simulink model "pixhawk_controller_position__ptCloud4_1"  (R2020a)
settings: Solver=ode4  StartTime=0.0  StopTime=30  FixedStep=0.01  RelTol=1e-3  EnableMultiTasking=on
InitFcn:
  | detector = load('ptOPDetector.mat');
  | OPdetector = detector.OPdetector;
undefined symbols (not defined in the file): g, Kd_p, Kd_q, Kd_r, Kd_vx, Kd_vy, Kd_vz, Kff_r, Kff_vx, Kff_vy, Kff_vz, Ki_p, Ki_q, Ki_r, Ki_vx, Ki_vy, Ki_vz, Kp_p, Kp_phi, Kp_psi, Kp_q, Kp_r, Kp_theta, Kp_vx, Kp_vy, Kp_vz, M, pointCloud_center, sigma_motor, w_h
libraries: visiontextngfix x1, sharedtransform x1, shared6dof x1, simulink_extras x1
(part 2 of 2)

== matlab function pixhawk_controller_position__ptCloud4_1/3D A* Algorithm/MATLAB Function8 ==
  data: octomap_center input; Obstacle output; pos_init input
function Obstacle = gen_3d_array(octomap_center,pos_init)

mapsize = [150 100 30];

Obstacle = int8(zeros(mapsize(1),mapsize(2),mapsize(3)));
grid_size = 0.2;
start_point = [pos_init(1) pos_init(2) pos_init(3)];

% align1 = int16(octomap_center/(grid_size)+0.5);
align1 = int16(octomap_center/(grid_size));
align2 = unique(align1,'rows');
align3 = [align2(:,1)+start_point(1) align2(:,2)+start_point(2) align2(:,3)+start_point(3)];

for i = 1:numel(align3)/3
    
    index_temp = align3(i,:);
    
    index_check = index_temp<3;
    if sum(index_check)>=1
        index_temp(index_check) = 3;
    end
    
    if index_temp(1) > mapsize(1)-2
        index_temp(1) = mapsize(1)-2;
    end
    if index_temp(2) > mapsize(2)-2
        index_temp(2) = mapsize(2)-2;
    end
    if index_temp(3) > mapsize(3)-2
        index_temp(3) = mapsize(3)-2;
    end
    

    index_x = index_temp(1)-1:index_temp(1)+1;
    index_y = index_temp(2)-1:index_temp(2)+1;
    index_z = index_temp(3)-1:index_temp(3)+1;

    Obstacle(index_x,index_temp(2)+1,index_temp(3)+1) = 1;
    Obstacle(index_x,index_temp(2)+1,index_temp(3)) = 1;
    Obstacle(index_x,index_temp(2)+1,index_temp(3)-1) = 1;
    Obstacle(index_x,index_temp(2),index_temp(3)+1) = 1;
    Obstacle(index_x,index_temp(2),index_temp(3)) = 1;
    Obstacle(index_x,index_temp(2),index_temp(3)-1) = 1;
    Obstacle(index_x,index_temp(2)-1,index_temp(3)+1) = 1;
    Obstacle(index_x,index_temp(2)-1,index_temp(3)) = 1;
    Obstacle(index_x,index_temp(2)-1,index_temp(3)-1) = 1;
    
%     Obstacle(index_temp(1)+1,index_temp(2)+2,index_z) = 1;
%     Obstacle(index_temp(1)+1,index_temp(2)-2,index_z) = 1;
%     Obstacle(index_temp(1)+1,index_y,index_temp(3)+2) = 1;
%     Obstacle(index_temp(1)+1,index_y,index_temp(3)-2) = 1;
%     Obstacle(index_temp(1),index_temp(2)+2,index_z) = 1;
%     Obstacle(index_temp(1),index_temp(2)-2,index_z) = 1;
%     Obstacle(index_temp(1),index_y,index_temp(3)+2) = 1;
%     Obstacle(index_temp(1),index_y,index_temp(3)-2) = 1;
%     Obstacle(index_temp(1)-1,index_temp(2)+2,index_z) = 1;
%     Obstacle(index_temp(1)-1,index_temp(2)-2,index_z) = 1;
%     Obstacle(index_temp(1)-1,index_y,index_temp(3)+2) = 1;
%     Obstacle(index_temp(1)-1,index_y,index_temp(3)-2) = 1;
    
    
    
    
%     Obstacle(index_temp(1)+2,index_temp(2)+2,index_z) = 1;
%     Obstacle(index_temp(1)+2,index_temp(2)+1,index_z) = 1;
%     Obstacle(index_temp(1)+2,index_temp(2),index_z) = 1;
%     Obstacle(index_temp(1)+2,index_temp(2)-1,index_z) = 1;
%     Obstacle(index_temp(1)+2,index_temp(2)-2,index_z) = 1;
%     
%     Obstacle(index_temp(1)+1,index_temp(2)+2,index_z) = 1;
%     Obstacle(index_temp(1)+1,index_temp(2)+1,index_z) = 1;
%     Obstacle(index_temp(1)+1,index_temp(2),index_z) = 1;
%     Obstacle(index_temp(1)+1,index_temp(2)-1,index_z) = 1;
%     Obstacle(index_temp(1)+1,index_temp(2)-2,index_z) = 1;
%     
%     Obstacle(index_temp(1),index_temp(2)+2,index_z) = 1;
%     Obstacle(index_temp(1),index_temp(2)+1,index_z) = 1;
%     Obstacle(index_temp(1),index_temp(2),index_z) = 1;
%     Obstacle(index_temp(1),index_temp(2)-1,index_z) = 1;
%     Obstacle(index_temp(1),index_temp(2)-2,index_z) = 1;
%     
%     Obstacle(index_temp(1)-1,index_temp(2)+2,index_z) = 1;
%     Obstacle(index_temp(1)-1,index_temp(2)+1,index_z) = 1;
%     Obstacle(index_temp(1)-1,index_temp(2),index_z) = 1;
%     Obstacle(index_temp(1)-1,index_temp(2)-1,index_z) = 1;
%     Obstacle(index_temp(1)-1,index_temp(2)-2,index_z) = 1;
%     
%     Obstacle(index_temp(1)-2,index_temp(2)+2,index_z) = 1;
%     Obstacle(index_temp(1)-2,index_temp(2)+1,index_z) = 1;
%     Obstacle(index_temp(1)-2,index_temp(2),index_z) = 1;
%     Obstacle(index_temp(1)-2,index_temp(2)-1,index_z) = 1;
%     Obstacle(index_temp(1)-2,index_temp(2)-2,index_z) = 1;
    
end

Obstacle(1:3,:,:)=1;
Obstacle(mapsize(1)-2:mapsize(1),:,:) = 1;
Obstacle(:,1:3,:) = 1;
Obstacle(:,mapsize(2)-2:mapsize(2),:) = 1;
Obstacle(:,:,1:3) = 1;
Obstacle(:,:,mapsize(3)-10:mapsize(3)) = 1;

end

== matlab function pixhawk_controller_position__ptCloud4_1/Path Guidance/MATLAB Function ==
  data: X_vel_cmd output; Y_vel_cmd output; odom input; Z_vel_cmd output; optimal_path_x input size=[128 1]; optimal_path_y input size=[128 1]; optimal_path_z input size=[128 1]; yaw_cmd output
function [X_vel_cmd,Y_vel_cmd,Z_vel_cmd,yaw_cmd] = fcn(odom,optimal_path_x,optimal_path_y,optimal_path_z)

P_gain = 0.5;

path_length = length(optimal_path_x);
K = inf(path_length,1);
optimal_path_norm = inf(path_length,3);

% optimal_path_x_temp = optimal_path_x.Data';
% optimal_path_y_temp = optimal_path_y.Data';

optimal_path_norm(:,1) = single(optimal_path_x - odom(1));
optimal_path_norm(:,2) = single(optimal_path_y - odom(2));
optimal_path_norm(:,3) = single(optimal_path_z - odom(3));

% optimal_path = [optimal_path_x' optimal_path_y'];
% optimal_path_norm = optimal_path - [odom(1) odom(2)];

for i=1:path_length
    K(i) = norm(optimal_path_norm(i,:));
end

[~,m] = min(K);



% Z_cmd = optimal_path_z(m);
if m >= 128
    m = 127;
end
% Z_cmd = optimal_path_z(m+1) + APF_vector(3);         % prediction
% X_cmd = optimal_path_x(m+1) + APF_vector(1);
% Y_cmd = optimal_path_y(m+1) + APF_vector(2);
Z_cmd = optimal_path_z(m+1);       
X_cmd = optimal_path_x(m+1);
Y_cmd = optimal_path_y(m+1);

error_z = (Z_cmd - odom(3));
error_x = (X_cmd - odom(1));
error_y = (Y_cmd - odom(2));

Z_vel_cmd = double(error_z*P_gain);
X_vel_cmd = double(error_x*P_gain);
Y_vel_cmd = double(error_y*P_gain);
% yaw_cmd = atan2(Y_cmd-odom(2),X_cmd-odom(1));        % 고쳐야함 
% yaw_cmd = atan2(optimal_path_y(m+1)-odom(2),optimal_path_x(m+1)-odom(1)); 
if m <= 125
    yaw_vector1 = [optimal_path_x(m+1)-odom(1) optimal_path_y(m+1)-odom(2)] / norm([optimal_path_x(m+1)-odom(1) optimal_path_y(m+1)-odom(2)]);
    yaw_vector2 = [optimal_path_x(m+2)-odom(1) optimal_path_y(m+2)-odom(2)] / norm([optimal_path_x(m+2)-odom(1) optimal_path_y(m+2)-odom(2)]);
    yaw_vector3 = [optimal_path_x(m+3)-odom(1) optimal_path_y(m+3)-odom(2)] / norm([optimal_path_x(m+3)-odom(1) optimal_path_y(m+3)-odom(2)]);
    yaw_vector = yaw_vector1 + yaw_vector2 + yaw_vector3;
    yaw_cmd = double( atan2(yaw_vector(2),yaw_vector(1)) );
%     yaw_cmd = double( ( atan2(optimal_path_y(m+1)-odom(2),optimal_path_x(m+1)-odom(1)) + atan2(optimal_path_y(m+2)-odom(2),optimal_path_x(m+2)-odom(1)) + atan2(optimal_path_y(m+3)-odom(2),optimal_path_x(m+3)-odom(1)) ) / 3 );
else
    yaw_cmd = 0;
end

end

== matlab function pixhawk_controller_position__ptCloud4_1/Generation_Angle_error/Attitude Generation (phi,theta,psi) ==
  data: DCM input; acc_cmd input; angle_error output; R_rp_x output
function [angle_error,R_rp_x]  = fcn(DCM,acc_cmd)
%#codegen

R_z           = DCM(3,:)'; 

% for i = 1:length(R_z)
%     if abs(R_z(i)) < 0.001
%         R_z(i) = 0;
%     end
% end

acc_unit      = R_z     / norm(R_z);
acc_cmd_unit  = acc_cmd / norm(acc_cmd);

angle_error = DCM * cross(acc_unit,acc_cmd_unit); %% e_R , consider phi, theta


% Calculate R_rp_x
angle = atan(norm(cross(acc_unit,acc_cmd_unit))/norm(dot(acc_unit,acc_cmd_unit))); % only phi,theta

e_R = angle_error;
R= DCM';

% e_R_cp matrix cross product
e_R_cp = zeros(3,3);
e_R_cp(1,2) = -e_R(3);
e_R_cp(1,3) =  e_R(2);
e_R_cp(2,1) =  e_R(3);
e_R_cp(2,3) = -e_R(1);
e_R_cp(3,1) = -e_R(2);
e_R_cp(3,2) =  e_R(1);

% Result
R_rp = R*(eye(3,3) + e_R_cp*sin(angle) + e_R_cp*e_R_cp*(1-cos(angle)));
R_rp_x = R_rp(:,1);
% acc_cmd_result = R_rp(:,3);

== matlab function pixhawk_controller_position__ptCloud4_1/Motor_Dynamics/Motor Dynamics/Motor Rotation Speed Generation ==
  data: w_dot_cmd input; w_state input; w_motor output; T_require output; Moment output; w_motor_square output; a_cmd input; DCM input
function [w_motor,T_require,Moment,w_motor_square] = fcn(w_dot_cmd,w_state,a_cmd,DCM)

w_motor        = zeros(4,1);
% ============= Quadrotor Spec  ==========================================%
kafa_f = 6.41*10^-6;                    % thrust coefficient
kafa_tau = 1.69*10^-2;                  % moment coefficient

L = 0.22/2;                               % length ( motor to motor) [m]
M = 0.5 ; %mass    [Kg]

I_T = [3.2*10^-3,3.2*10^-3,5.5*10^-3];  % total moment
I_P = [0,0,1.5*10^-5];                  % propeller reaction moment
I_B = I_T - 4*I_P;                      % frame inertia moment
Inertia = diag(I_B);
% 
% T_require = M * norm(a_cmd);
T_hover = [0,0,1]; %Thrust
R_z = DCM(:,3);
g = 9.8; %gravity [m/s^2]
T_require = M*(abs(a_cmd) / dot(T_hover,R_z));


Moment = Inertia*w_dot_cmd + cross(w_state,Inertia*w_state);

A = [1       ,  1         ,   1         ,   1;
    0        ,  L         ,   0         ,  -L;
    -L       ,  0         ,   L         ,   0;
    kafa_tau , -kafa_tau  ,   kafa_tau  ,  -kafa_tau];

w_motor_square = A^-1 * [T_require;Moment]/kafa_f;

for i = 1:length(w_motor_square)
    w_motor(i) = sqrt(abs(w_motor_square(i)));
end

== matlab function pixhawk_controller_position__ptCloud4_1/Quadrotor Dynamics/중력항 고려 ==
  data: Mg input; DCM_e2b input; Fe output
function Fe = fcn(Mg,DCM_e2b)

Fe=DCM_e2b*Mg;

== matlab function pixhawk_controller_position__ptCloud4_1/Generation_Angle_error/Attitude Generation(psi^*) ==
  data: R_rp_x input; acc_cmd input; Bearing_angle input; psi_angle_error output
function psi_angle_error   = fcn(R_rp_x,acc_cmd,Bearing_angle)
%#codegen

acc_cmd_unit  = acc_cmd / norm(acc_cmd); % define hat(k)_B_des
sigma = Bearing_angle;

j_sigma_des = [-sin(sigma),cos(sigma),0]; % hat(i)_sigma_des

i_B_des =  cross(j_sigma_des,acc_cmd_unit);
R_sp_x  =  i_B_des;
% 
% temp  = cross(R_rp_x,R_sp_x);
% temp2 = dot(R_rp_x,R_sp_x);

psi_angle_error = atan(cross(R_rp_x,R_sp_x)*acc_cmd_unit/dot(R_rp_x,R_sp_x))*acc_cmd_unit(3)^2;

% psi_angle_error = atan(norm(cross(R_rp_x,R_sp_x))/dot(R_rp_x,R_sp_x));

== matlab function pixhawk_controller_position__ptCloud4_1/Generation_Angle_error/Attitude Generation(phi,theta,psi^*) ==
  data: angle_error input; psi_angle_error input; angle_error_result output
function angle_error_result  = fcn(angle_error,psi_angle_error)
%#codegen

angle_error_result = [angle_error(1);angle_error(2);psi_angle_error];

% if norm(temp) ~= 0
%     angle_error_result  = temp / norm(temp);
% else
%     angle_error_result  = temp;
% end

== matlab function pixhawk_controller_position__ptCloud4_1/MATLAB Function ==
  settings: updateMethod=DISCRETE
  data: current_pos input; pointCloud_current output size=[50000 3]; pointCloud_center input
function pointCloud_current = fcn(current_pos, pointCloud_center)

persistent pointCloud_old block_hz
if isempty(block_hz)
    block_hz = 5;
end
pointCloud_center = double(pointCloud_center);

size_max = 50000;

pointCloud_new = nan(size_max,3);
pointCloud_current = nan(size_max,3);

% if block_hz ==5
%     block_hz = 0;
    for aaa = 1:numel(pointCloud_center)/3
        if sqrt((pointCloud_center(aaa,1)-current_pos(1))^2+(pointCloud_center(aaa,2)-current_pos(2))^2+(pointCloud_center(aaa,3)-current_pos(3))^2)<4
            %         pointCloud_new = cat(1,pointCloud_new,pointCloud_center(aaa,:));
            pointCloud_new(aaa,:) = pointCloud_center(aaa,:);
        end
    end
    
    if isempty(pointCloud_old)
        pointCloud_old = nan(size_max,3);
    end
    
    pointCloud_temp=cat(1,rmmissing(pointCloud_old),rmmissing(pointCloud_new));
    pointCloud_unique = unique(pointCloud_temp,'rows');
    % pointCloud_current=cat(1,cat(1,rmmissing(pointCloud_old),rmmissing(pointCloud_new)),nan(100000-(numel(rmmissing(pointCloud_old))/3+numel(rmmissing(pointCloud_new))/3),3));
    % pointCloud_current=[rmmissing(pointCloud_temp);nan(200000-numel(rmmissing(pointCloud_temp))/3,3)];
    for aaa = 1:numel(pointCloud_unique)/3
        if (~isnan(pointCloud_unique(aaa,1)))&&(~isnan(pointCloud_unique(aaa,2)))&&(~isnan(pointCloud_unique(aaa,3)))
            pointCloud_current(aaa,:)=pointCloud_unique(aaa,:);
        end
    end
    
    
% end

pointCloud_old = pointCloud_current;
% block_hz = block_hz +1;

== matlab function pixhawk_controller_position__ptCloud4_1/Quadrotor Dynamics/Translation body -> Earth ==
  data: Ab input; DCM input; Ae output
function Ae = fcn(Ab,DCM)
%#codegen

ax_b = Ab(1);
ay_b = Ab(2);
az_b = Ab(3);

a_b = [ax_b;ay_b;az_b];
Ae = DCM'*a_b;

== matlab function pixhawk_controller_position__ptCloud4_1/Position_Controller/Velocity Controller/Acceleration Saturation ==
  data: a_cmd input; a_cmd_sat output; a_norm output
function [a_cmd_sat,a_norm] = fcn(a_cmd)
%#codegen

tilt_max = 35*pi/180; % [rad  ] , tolerant tilt , user define
thr_max  = 11;        % [m/s^2] , tolerant acceleration , user define (90% maximum, 50% hovering)
% thr_max  = 9.8/50 * 90; 

thrust_sp_xy_len = norm([a_cmd(1) a_cmd(2)]);
thrust_xy_max    = abs(a_cmd(3)) * tan(tilt_max);

if thrust_sp_xy_len >= thrust_xy_max
    k =  thrust_xy_max/thrust_sp_xy_len;
    a_cmd_sat = [a_cmd(1)*k ; a_cmd(2)*k ; a_cmd(3)];
else
    a_cmd_sat = a_cmd;
end


if a_cmd_sat(3)/abs(a_cmd_sat(3)) >= 0 
    if abs(a_cmd_sat(3)) >= thr_max

        k  = a_cmd_sat(3) / abs(a_cmd_sat(3));
        a_cmd_sat = [0 ; 0 ; k*thr_max];
    else
        thrust_sp_xy_len_sat = sqrt(a_cmd_sat(1)^2 + a_cmd_sat(2)^2);
        thrust_xy_max_sat    = sqrt(-a_cmd_sat(3)^2 + thr_max^2); 

        if thrust_sp_xy_len_sat >= thrust_xy_max_sat
            k = thrust_xy_max_sat / thrust_sp_xy_len_sat;
            a_cmd_sat = [a_cmd_sat(1)*k ; a_cmd_sat(2)*k ; a_cmd_sat(3)];
        end
    end
else
    a_cmd_sat = [a_cmd_sat(1) ; a_cmd_sat(2) ; 0.00001];
end

a_norm = norm(a_cmd_sat);

== matlab function pixhawk_controller_position__ptCloud4_1/Path Guidance/MATLAB Function1 ==
  data: w input; yaw output; x input; y input; z input
function yaw = quat2yaw(w,x,y,z)

euler_angle = quat2eul([w x y z],'ZYX');
yaw = euler_angle(1);
end
